simulink model "DA40_Flight_Model"  (R2023a)
settings: Solver=FixedStepAuto  StartTime=Start_Time  StopTime=End_Time  FixedStep=Time_Step  RelTol=1e-3
undefined symbols (not defined in the file or in its folder): BSFC_LUT, dayofyear, Earth, Initial_X, lookaheadDist, PowerFactor_LUT, STGeometry, Vehicle, waypoints, WGS84
libraries: slpidlib x8, simulink_extras x3, aerolibatmos2 x2, mspsensorlib x2, aerolibtransform2 x2, simulink x1, aerolibwind2 x1, uavalgslib x1
(part 2 of 3)

== system DA40_Flight_Model/Truth Model/Control/Subsystem4 ==
  Reference : Inport
  States : Inport  Port=2
  Display : Display
  Display1 : Display
  Display2 : Display
  PID Controller (2DOF) : slpidlib/PID Controller (2DOF)  Controller=PID  Form=Parallel  TimeDomain=Continuous-time  UseExternalTs=off  SampleTime=-1  IntegratorMethod=Forward Euler  FilterMethod=Forward Euler  ControllerParametersSource=internal  P=0  I=1  UseKiTs=off  D=0  N=100  UseFilter=on  b=1  c=1  TunerSelectOption=Transfer Function Based (PID Tuner App)  InitialConditionSource=internal  InitialConditionForIntegrator=0  InitialConditionForFilter=0  DifferentiatorICPrevScaledInput=0  ExternalReset=none  TrackingMode=off  Kt=1  LimitOutput=on  SatLimitsSource=internal  UpperSaturationLimit=1  LowerSaturationLimit=0  LinearizeAsGain=on  AntiWindupMode=none  Kb=1  LimitIntegrator=off  UpperIntegratorSaturationLimit=inf  LowerIntegratorSaturationLimit=-inf  POutMin=[]  POutMax=[]  IOutMin=[]  IOutMax=[]  DOutMin=[]  DOutMax=[]  NOutMin=[]  NOutMax=[]  bOutMin=[]  bOutMax=[]  cOutMin=[]  cOutMax=[]  SumOutMin=[]  SumOutMax=[]  SaturationOutMin=[]  SaturationOutMax=[]  PParamMin=[]  PParamMax=[]  IParamMin=[]  IParamMax=[]  DParamMin=[]  DParamMax=[]  NParamMin=[]  NParamMax=[]  bParamMin=[]  bParamMax=[]  cParamMin=[]  cParamMax=[]  KbParamMin=[]  KbParamMax=[]  KtParamMin=[]  KtParamMax=[]  KbOutMin=[]  KbOutMax=[]  KtOutMin=[]  KtOutMax=[]  IntegratorOutMin=[]  IntegratorOutMax=[]  FilterOutMin=[]  FilterOutMax=[]  SumI1OutMin=[]  SumI1OutMax=[]  SumI2OutMin=[]  SumI2OutMax=[]  SumI3OutMin=[]  SumI3OutMax=[]  SumI4OutMin=[]  SumI4OutMax=[]  SumDOutMin=[]  SumDOutMax=[]  Sum1OutMin=[]  Sum1OutMax=[]  Sum2OutMin=[]  Sum2OutMax=[]  Sum3OutMin=[]  Sum3OutMax=[]  DifferentiatorOutMin=[]  DifferentiatorOutMax=[]  FilterDiffOutCoefMin=[]  FilterDiffOutCoefMax=[]  ReciprocalOutMin=[]  ReciprocalOutMax=[]  SumDenOutMin=[]  SumDenOutMax=[]  SumNumOutMin=[]  SumNumOutMax=[]  DivideOutMin=[]  DivideOutMax=[]  UdiffTsProdOutMin=[]  UdiffTsProdOutMax=[]  NTsProdOutMin=[]  NTsProdOutMax=[]  UintegralTsProdOutMin=[]  UintegralTsProdOutMax=[]  UngainTsProdOutMin=[]  UngainTsProdOutMax=[]  ClampingZeroOutDataTypeStr=Inherit: Inherit via back propagation  ClampingZeroOutMin=[]  ClampingZeroOutMax=[]  FilterDenConstantOutDataTypeStr=Inherit: Inherit via back propagation  FilterDenConstantOutMin=[]  FilterDenConstantOutMax=[]  PCopyOutDataTypeStr=Inherit: Inherit via back propagation  PCopyOutMin=[]  PCopyOutMax=[]  NCopyOutDataTypeStr=Inherit: Inherit via back propagation  NCopyOutMin=[]  NCopyOutMax=[]  IntegratorContinuousStateAttributes=''  IntegratorStateMustResolveToSignalObject=off  IntegratorRTWStateStorageClass=Auto  FilterContinuousStateAttributes=''  FilterStateMustResolveToSignalObject=off  FilterRTWStateStorageClass=Auto  ParallelPVariant=InternalParameters  IdealPVariant=Disabled  IVariant=InternalParameters  DVariant=InternalParameters  bVariant=InternalParameters  cVariant=InternalParameters  IntegratorVariant=Continuous  SatVariant=Enabled  AWVariant=Passthrough  PCopyVariant=Disabled  TRVariant=Disabled  FdbkBlocksVariant=Forward  IdealPFdbkVariant=Disabled  SatFdbkVariant=Disabled  DerivativeFilterVariant=ContFilter  NVariant=InternalParameters  NCopyVariant=Disabled  FilterICVariant=InternalICsFilter  IntegratorICVariant=InternalICs  ExternalResetVariant=Disabled  TRSumVariant=Passthrough  SumFdbkVariant=Disabled  SumVariant=Sum_PID  TsampFilterVariant=InternalTs  TsampNgainVariant=Passthrough  TsampIntegralVariant=Disabled_SignalSpec  ExternalSaturationOutDataTypeStr=Inherit: Same as second input
  Out1 : Outport
  " " : Outport  Port=2
  wires:
  PID Controller (2DOF)/1 -> Display2/1, Out1/1
  [truepropEff] -> Display/1, PID Controller (2DOF)/2
  Reference/1 -> Display1/1, PID Controller (2DOF)/1
  States/1 -> " "/1

== system DA40_Flight_Model/Truth Model/Control/Subsystem5 ==
  Reference : Inport
  States : Inport  Port=2
  Out1 : Outport
  " " : Outport  Port=2
  wires:
  Reference/1 -> Out1/1
  States/1 -> " "/1

== system DA40_Flight_Model/Truth Model/Control/Subsystem6 ==
  Reference : Inport
  States : Inport  Port=2
  Out1 : Outport
  " " : Outport  Port=2
  wires:
  Reference/1 -> Out1/1
  States/1 -> " "/1

== system DA40_Flight_Model/Truth Model/Control/Subsystem7 ==
  Reference : Inport
  States : Inport  Port=2
  Out1 : Outport
  " " : Outport  Port=2
  wires:
  Reference/1 -> Out1/1
  States/1 -> " "/1

== system DA40_Flight_Model/Truth Model/Control/Subsystem8 ==
  Reference : Inport
  States : Inport  Port=2
  Out1 : Outport
  " " : Outport  Port=2
  wires:
  Reference/1 -> Out1/1
  States/1 -> " "/1

== system DA40_Flight_Model/Truth Model/Control/Subsystem9 ==
  Reference : Inport
  States : Inport  Port=2
  Out1 : Outport
  " " : Outport  Port=2
  wires:
  States/1 -> " "/1
  Reference/1 -> Out1/1

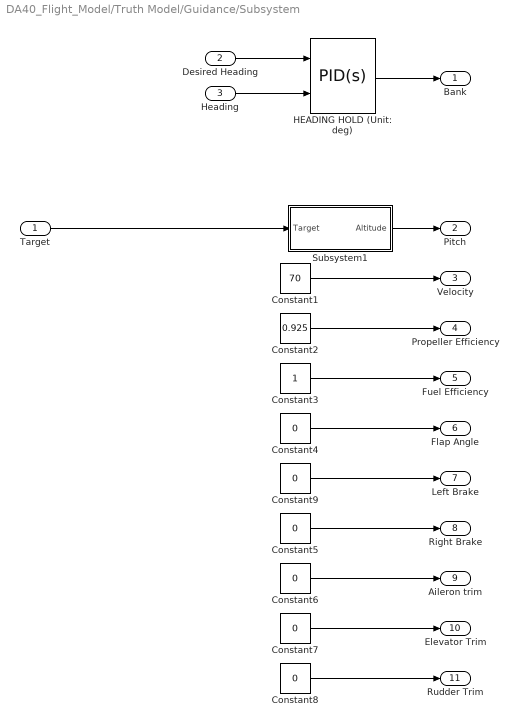
== system DA40_Flight_Model/Truth Model/Guidance/Subsystem ==
  Target : Inport
  Desired Heading : Inport  Port=2
  Heading : Inport  Port=3
  Constant1 : Constant  Value=70
  Constant2 : Constant  Value=0.925
  Constant3 : Constant
  Constant{4..9} (6 alike) : Constant  Value=0
  HEADING HOLD (Unit: deg) : slpidlib/PID Controller (2DOF)  Controller=PID  Form=Parallel  TimeDomain=Continuous-time  UseExternalTs=off  SampleTime=-1  IntegratorMethod=Forward Euler  FilterMethod=Forward Euler  ControllerParametersSource=internal  P=1  I=0.001  UseKiTs=off  D=0  N=100  UseFilter=on  b=1  c=0  TunerSelectOption=Transfer Function Based (PID Tuner App)  InitialConditionSource=internal  InitialConditionForIntegrator=0  InitialConditionForFilter=0  DifferentiatorICPrevScaledInput=0  ExternalReset=none  TrackingMode=off  Kt=1  LimitOutput=on  SatLimitsSource=internal  UpperSaturationLimit=30  LowerSaturationLimit=-30  LinearizeAsGain=on  AntiWindupMode=clamping  Kb=1  LimitIntegrator=off  UpperIntegratorSaturationLimit=inf  LowerIntegratorSaturationLimit=-inf  POutMin=[]  POutMax=[]  IOutMin=[]  IOutMax=[]  DOutMin=[]  DOutMax=[]  NOutMin=[]  NOutMax=[]  bOutMin=[]  bOutMax=[]  cOutMin=[]  cOutMax=[]  SumOutMin=[]  SumOutMax=[]  SaturationOutMin=[]  SaturationOutMax=[]  PParamMin=[]  PParamMax=[]  IParamMin=[]  IParamMax=[]  DParamMin=[]  DParamMax=[]  NParamMin=[]  NParamMax=[]  bParamMin=[]  bParamMax=[]  cParamMin=[]  cParamMax=[]  KbParamMin=[]  KbParamMax=[]  KtParamMin=[]  KtParamMax=[]  KbOutMin=[]  KbOutMax=[]  KtOutMin=[]  KtOutMax=[]  IntegratorOutMin=[]  IntegratorOutMax=[]  FilterOutMin=[]  FilterOutMax=[]  SumI1OutMin=[]  SumI1OutMax=[]  SumI2OutMin=[]  SumI2OutMax=[]  SumI3OutMin=[]  SumI3OutMax=[]  SumI4OutMin=[]  SumI4OutMax=[]  SumDOutMin=[]  SumDOutMax=[]  Sum1OutMin=[]  Sum1OutMax=[]  Sum2OutMin=[]  Sum2OutMax=[]  Sum3OutMin=[]  Sum3OutMax=[]  DifferentiatorOutMin=[]  DifferentiatorOutMax=[]  FilterDiffOutCoefMin=[]  FilterDiffOutCoefMax=[]  ReciprocalOutMin=[]  ReciprocalOutMax=[]  SumDenOutMin=[]  SumDenOutMax=[]  SumNumOutMin=[]  SumNumOutMax=[]  DivideOutMin=[]  DivideOutMax=[]  UdiffTsProdOutMin=[]  UdiffTsProdOutMax=[]  NTsProdOutMin=[]  NTsProdOutMax=[]  UintegralTsProdOutMin=[]  UintegralTsProdOutMax=[]  UngainTsProdOutMin=[]  UngainTsProdOutMax=[]  ClampingZeroOutDataTypeStr=Inherit: Inherit via back propagation  ClampingZeroOutMin=[]  ClampingZeroOutMax=[]  FilterDenConstantOutDataTypeStr=Inherit: Inherit via back propagation  FilterDenConstantOutMin=[]  FilterDenConstantOutMax=[]  PCopyOutDataTypeStr=Inherit: Inherit via back propagation  PCopyOutMin=[]  PCopyOutMax=[]  NCopyOutDataTypeStr=Inherit: Inherit via back propagation  NCopyOutMin=[]  NCopyOutMax=[]  IntegratorContinuousStateAttributes=''  IntegratorStateMustResolveToSignalObject=off  IntegratorRTWStateStorageClass=Auto  FilterContinuousStateAttributes=''  FilterStateMustResolveToSignalObject=off  FilterRTWStateStorageClass=Auto  ParallelPVariant=InternalParameters  IdealPVariant=Disabled  IVariant=InternalParameters  DVariant=InternalParameters  bVariant=InternalParameters  cVariant=InternalParameters  IntegratorVariant=Continuous  SatVariant=Enabled  AWVariant=ContClampingParallel  PCopyVariant=Disabled  TRVariant=Disabled  FdbkBlocksVariant=Forward  IdealPFdbkVariant=Disabled  SatFdbkVariant=Disabled  DerivativeFilterVariant=ContFilter  NVariant=InternalParameters  NCopyVariant=Disabled  FilterICVariant=InternalICsFilter  IntegratorICVariant=InternalICs  ExternalResetVariant=Disabled  TRSumVariant=Passthrough  SumFdbkVariant=Disabled  SumVariant=Sum_PID  TsampFilterVariant=InternalTs  TsampNgainVariant=Passthrough  TsampIntegralVariant=Disabled_SignalSpec  ExternalSaturationOutDataTypeStr=Inherit: Same as second input
  Subsystem1 : Subsystem
  Bank : Outport
  Pitch : Outport  Port=2
  Velocity : Outport  Port=3
  Propeller Efficiency : Outport  Port=4
  Fuel Efficiency : Outport  Port=5
  Flap Angle : Outport  Port=6
  Left Brake : Outport  Port=7
  Right Brake : Outport  Port=8
  Aileron trim : Outport  Port=9
  Elevator Trim : Outport  Port=10
  Rudder Trim : Outport  Port=11
  wires:
  Subsystem1/1(Altitude) -> Pitch/1
  Constant1/1 -> Velocity/1
  Constant2/1 -> Propeller Efficiency/1
  Constant3/1 -> Fuel Efficiency/1
  Constant4/1 -> Flap Angle/1
  Constant9/1 -> Left Brake/1
  Constant5/1 -> Right Brake/1
  Constant6/1 -> Aileron trim/1
  Constant7/1 -> Elevator Trim/1
  Constant8/1 -> Rudder Trim/1
  Desired Heading/1 -> HEADING HOLD (Unit: deg)/1
  Target/1 -> Subsystem1/1(Target)
  HEADING HOLD (Unit: deg)/1 -> Bank/1
  Heading/1 -> HEADING HOLD (Unit: deg)/2

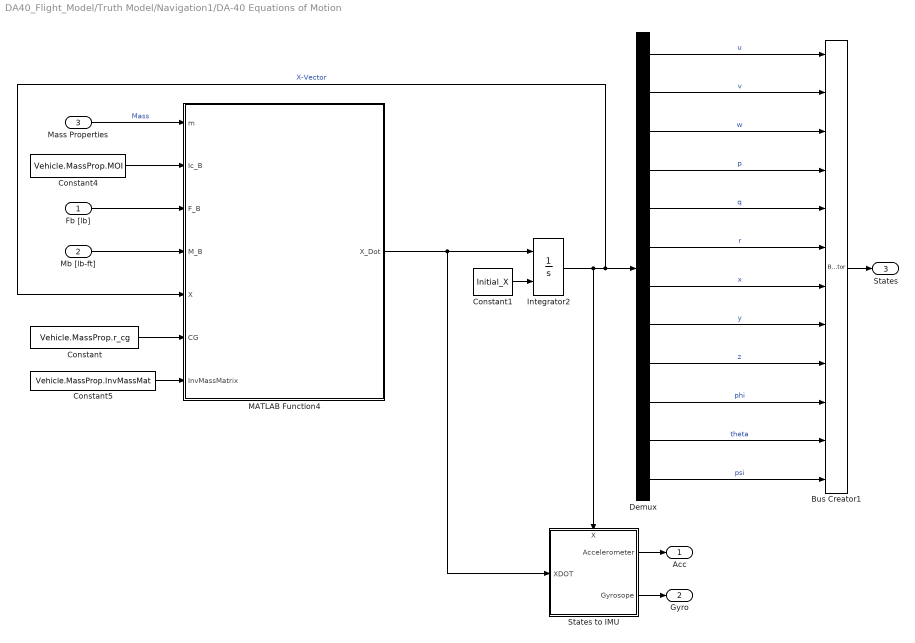
== system DA40_Flight_Model/Truth Model/Navigation1/DA-40 Equations of Motion ==
  Fb [lb] : Inport
  Mb [lb-ft] : Inport  Port=2
  Mass Properties : Inport  Port=3
  Bus Creator1 : BusCreator  Inputs=12
  Constant : Constant  Value=Vehicle.MassProp.r_cg
  Constant1 : Constant  Value=Initial_X
  Constant4 : Constant  Value=Vehicle.MassProp.MOI  VectorParams1D=off
  Constant5 : Constant  Value=Vehicle.MassProp.InvMassMat
  Demux : Demux  Outputs=12
  Integrator2 : Integrator  InitialConditionSource=external
  MATLAB Function4 : MATLAB Function  TreatAsAtomicUnit=on
  States to IMU : Subsystem
      settings: PortSchema="{\"entries\":[{\"content\":{\"sides\":[{\"content\":{\"connectorIds\":[\"In1\"]},\"type\":\"ConnectorPlacement.EquallySpacedRectSide\",\"uuid\":\"70ccec87-9e5d-4668-bab7-5e3830192650\"},{\"content\":{\"connectorIds\":[\"Out1\",\"Out2\"],\"side\":\"RIGHT\"},\"type\":\"ConnectorPlacement.EquallySpacedRectSide\",\"uuid\":\"cc9275bd-5621-4491-a3fb-001b77b42a94\"},{\"content\":{\"connectorIds\":[\"In2\"],\"side\":\"TOP\"},\"type\":\"ConnectorPlacement.EquallySpacedRectSide\",\"uuid\":\"9fc04c5e-8168-4117-852d-b94be052fe47\"}]},\"type\":\"ConnectorPlacement.EquallySpacedConnector\",\"uuid\":\"901299e0-db58-4c82-bff1-da00e9d52dc5\"}],\"packageUris\":[\"http://schema.mathworks.com/mf0/Connector/R2020b\"],\"version\":\"1.0\"}"
  Acc : Outport
  Gyro : Outport  Port=2
  States : Outport  Port=3
  wires:
  Mb [lb-ft]/1 -> MATLAB Function4/4(M_B)
  Fb [lb]/1 -> MATLAB Function4/3(F_B)
  Mass Properties/1 -> MATLAB Function4/1(m)  "Mass"
  Constant4/1 -> MATLAB Function4/2(Ic_B)
  Constant1/1 -> Integrator2/2
  Integrator2/1 -> States to IMU/2(X), MATLAB Function4/5(X), Demux/1  "X-Vector"
  Constant/1 -> MATLAB Function4/6(CG)
  Constant5/1 -> MATLAB Function4/7(InvMassMatrix)
  Demux/1 -> Bus Creator1/1  "u"
  Demux/2 -> Bus Creator1/2  "v"
  Demux/3 -> Bus Creator1/3  "w"
  Demux/4 -> Bus Creator1/4  "p"
  Demux/5 -> Bus Creator1/5  "q"
  Demux/6 -> Bus Creator1/6  "r"
  Demux/7 -> Bus Creator1/7  "x"
  Demux/8 -> Bus Creator1/8  "y"
  Demux/9 -> Bus Creator1/9  "z"
  Demux/10 -> Bus Creator1/10  "phi"
  Demux/11 -> Bus Creator1/11  "theta"
  Demux/12 -> Bus Creator1/12  "psi"
  MATLAB Function4/1(X_Dot) -> States to IMU/1(XDOT), Integrator2/1
  States to IMU/1(Accelerometer) -> Acc/1
  Bus Creator1/1 -> States/1
  States to IMU/2(Gyrosope) -> Gyro/1

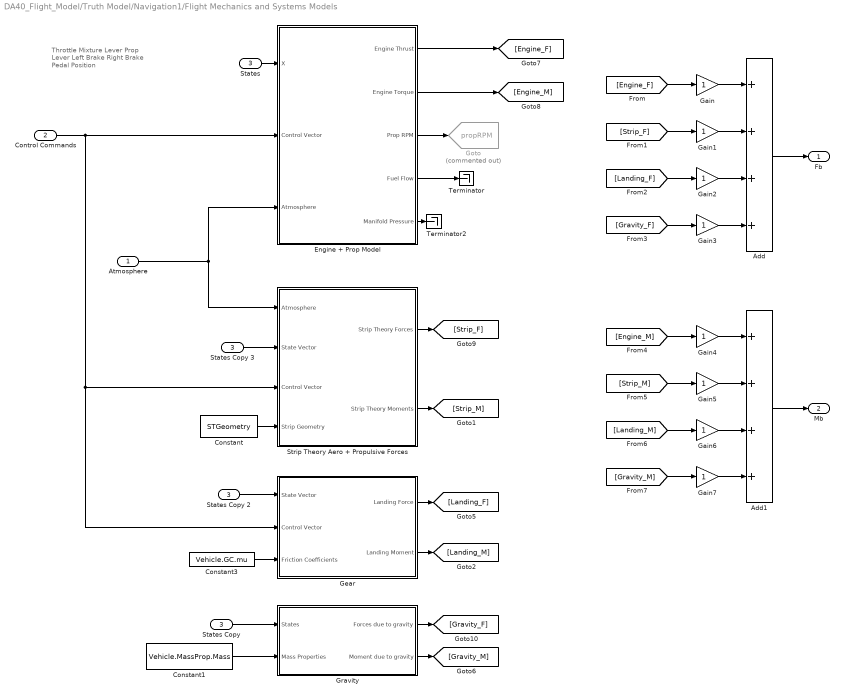
== system DA40_Flight_Model/Truth Model/Navigation1/Flight Mechanics and Systems Models ==
  note: Throttle
      | Mixture Lever
      | Prop Lever
      | Left Brake
      | Right Brake
      | Pedal Position
  Atmosphere : Inport
  Control Commands : Inport  Port=2
  States : Inport  Port=3
  Add : Sum  Inputs=++++
  Add1 : Sum  Inputs=++++
  Constant : Constant  Value=STGeometry
  Constant1 : Constant  Value=Vehicle.MassProp.Mass
  Constant3 : Constant  Value=Vehicle.GC.mu
  Engine + Prop Model : Subsystem
  Gain{,1..7} (8 alike) : Gain
  Gear : Subsystem
  Goto : Goto  Commented=on  GotoTag=propRPM  TagVisibility=global
  Gravity : Subsystem
  States Copy : InportShadow  Port=3
  States Copy 2 : InportShadow  Port=3
  States Copy 3 : InportShadow  Port=3
  Strip Theory Aero + Propulsive Forces : Subsystem
  Terminator : Terminator
  Terminator2 : Terminator
  Fb : Outport
  Mb : Outport  Port=2
  wires:
  States/1 -> Engine + Prop Model/1(X)
  Constant1/1 -> Gravity/2(Mass Properties)
  Constant/1 -> Strip Theory Aero + Propulsive Forces/4(Strip Geometry)
  Engine + Prop Model/5(Manifold Pressure) -> Terminator2/1
  Engine + Prop Model/3(Prop RPM) -> Goto/1
  Constant3/1 -> Gear/3(Friction Coefficients)
  Add1/1 -> Mb/1
  States Copy/1 -> Gravity/1(States)
  States Copy 2/1 -> Gear/1(State Vector)
  States Copy 3/1 -> Strip Theory Aero + Propulsive Forces/2(State Vector)
  Control Commands/1 -> Strip Theory Aero + Propulsive Forces/3(Control Vector), Gear/2(Control Vector), Engine + Prop Model/2(Control Vector)
  Engine + Prop Model/2(Engine Torque) -> [Engine_M]
  Strip Theory Aero + Propulsive Forces/2(Strip Theory Moments) -> [Strip_M]
  Gear/2(Landing Moment) -> [Landing_M]
  Gravity/2(Moment due to gravity) -> [Gravity_M]
  Gravity/1(Forces due to gravity) -> [Gravity_F]
  Gear/1(Landing Force) -> [Landing_F]
  Strip Theory Aero + Propulsive Forces/1(Strip Theory Forces) -> [Strip_F]
  Engine + Prop Model/1(Engine Thrust) -> [Engine_F]
  Add/1 -> Fb/1
  [Engine_F] -> Gain/1
  [Strip_F] -> Gain1/1
  [Landing_F] -> Gain2/1
  [Gravity_F] -> Gain3/1
  [Engine_M] -> Gain4/1
  [Strip_M] -> Gain5/1
  [Landing_M] -> Gain6/1
  [Gravity_M] -> Gain7/1
  Gain/1 -> Add/1
  Gain1/1 -> Add/2
  Gain2/1 -> Add/3
  Gain3/1 -> Add/4
  Gain4/1 -> Add1/1
  Gain5/1 -> Add1/2
  Gain6/1 -> Add1/3
  Gain7/1 -> Add1/4
  Atmosphere/1 -> Strip Theory Aero + Propulsive Forces/1(Atmosphere), Engine + Prop Model/3(Atmosphere)
  Engine + Prop Model/4(Fuel Flow) -> Terminator/1

== system DA40_Flight_Model/Noise Model/Navigation/DA-40 Equations of Motion/States to IMU ==
  XDOT : Inport
  X : Inport  Port=2
  IMU : mspsensorlib/IMU  DispRefFrame=NED  Temperature=25  MagneticFieldNED=[ 27.5550, -2.4169, -16.0849 ]  MagneticFieldENU=[ -2.4169, 27.5550, 16.0849 ]  SeedDouble=67  SimulateUsing=Code generation  AccelParamsMeasurementRange=Inf  AccelParamsResolution=0  AccelParamsConstantBias=[ 0, 0, 0 ]  AccelParamsAxesMisalignment=[ 100, 0, 0; 0, 100, 0; 0, 0, 100 ]  AccelParamsNoiseDensity=[ 0, 0, 0 ]  AccelParamsBiasInstability=[ 0, 0, 0 ]  AccelParamsRandomWalk=[ 0, 0, 0 ]  AccelParamsTemperatureBias=[ 0, 0, 0 ]  AccelParamsTemperatureScaleFactor=[ 0, 0, 0 ]  GyroParamsMeasurementRange=Inf  GyroParamsResolution=0  GyroParamsConstantBias=[ 0, 0, 0 ]  GyroParamsAxesMisalignment=[ 100, 0, 0; 0, 100, 0; 0, 0, 100 ]  GyroParamsAccelerationBias=[ 0, 0, 0 ]  GyroParamsNoiseDensity=[ 0, 0, 0 ]  GyroParamsBiasInstability=[ 0, 0, 0 ]  GyroParamsRandomWalk=[ 0, 0, 0 ]  GyroParamsTemperatureBias=[ 0, 0, 0 ]  GyroParamsTemperatureScaleFactor=[ 0, 0, 0 ]  MagParamsMeasurementRange=Inf  MagParamsResolution=0  MagParamsConstantBias=[ 0, 0, 0 ]  MagParamsAxesMisalignment=[ 100, 0, 0; 0, 100, 0; 0, 0, 100 ]  MagParamsNoiseDensity=[ 0, 0, 0 ]  MagParamsBiasInstability=[ 0, 0, 0 ]  MagParamsRandomWalk=[ 0, 0, 0 ]  MagParamsTemperatureBias=[ 0, 0, 0 ]  MagParamsTemperatureScaleFactor=[ 0, 0, 0 ]
  MATLAB Function : MATLAB Function  TreatAsAtomicUnit=on
  Rate Transition : RateTransition
  Rate Transition1 : RateTransition
  Rate Transition2 : RateTransition
  Terminator : Terminator
  Accelerometer : Outport
  Gyrosope : Outport  Port=2
  wires:
  IMU/3 -> Terminator/1
  IMU/2 -> Gyrosope/1
  IMU/1 -> Accelerometer/1
  X/1 -> MATLAB Function/1(X)
  XDOT/1 -> MATLAB Function/2(XDOT)
  MATLAB Function/1(ACC) -> Rate Transition2/1
  MATLAB Function/2(GYRO) -> Rate Transition1/1
  MATLAB Function/3(DCMBN) -> Rate Transition/1
  Rate Transition/1 -> IMU/3
  Rate Transition1/1 -> IMU/2
  Rate Transition2/1 -> IMU/1

== system DA40_Flight_Model/Noise Model/Navigation/Flight Mechanics and Systems Models/Engine + Prop Model ==
  X : Inport
  Control Vector : Inport  Port=2
  Atmosphere : Inport  Port=3
  Bus Selector : BusSelector  OutputSignals=Throttle,Mixture Lever,Prop Lever
  Subsystem : Subsystem
  Engine Thrust : Outport
  Engine Torque : Outport  Port=2
  Prop RPM : Outport  Port=3  PortDimensions=1
  Fuel Flow : Outport  Port=4  PortDimensions=1
  Manifold Pressure : Outport  Port=5  PortDimensions=1
  wires:
  X/1 -> Subsystem/1(X)
  Subsystem/3(Prop RPM) -> Prop RPM/1
  Subsystem/4(Fuel Flow) -> Fuel Flow/1
  Subsystem/5(Manifold Pressure) -> Manifold Pressure/1
  Control Vector/1 -> Bus Selector/1
  Bus Selector/1 -> Subsystem/2(Throttle Setting)  "<Throttle>"
  Bus Selector/2 -> Subsystem/3(Mix)  "<Mixture Lever>"
  Bus Selector/3 -> Subsystem/4(Prop Pitch)  "<Prop Lever>"
  Atmosphere/1 -> Subsystem/5(Atmosphere)
  Subsystem/2(Engine Torque) -> Engine Torque/1
  Subsystem/1(Engine Thrust) -> Engine Thrust/1

== system DA40_Flight_Model/Noise Model/Navigation/Flight Mechanics and Systems Models/Gear ==
  State Vector : Inport
  Control Vector : Inport  Port=2
  Friction Coefficients : Inport  Port=3
  " " : MATLAB Function  TreatAsAtomicUnit=on
  Bus Selector : BusSelector  OutputSignals=LeftBrake,RightBrake,Pedal Posn
  Mux : Mux  Inputs=3
  Landing Force : Outport
  Landing Moment : Outport  Port=2
  wires:
  Friction Coefficients/1 -> " "/3(mu)
  State Vector/1 -> " "/2(X)
  " "/1(Ground_Forces) -> Landing Force/1
  " "/2(Ground_Moments) -> Landing Moment/1
  Control Vector/1 -> Bus Selector/1
  Mux/1 -> " "/1(U)
  Bus Selector/1 -> Mux/1  "<LeftBrake>"
  Bus Selector/2 -> Mux/2  "<RightBrake>"
  Bus Selector/3 -> Mux/3  "<Pedal Posn>"

== system DA40_Flight_Model/Noise Model/Navigation/Flight Mechanics and Systems Models/Gravity ==
  States : Inport
  Mass Properties : Inport  Port=2
  Constant : Constant  Value=Vehicle.MassProp.r_cg
  MATLAB Function : MATLAB Function  TreatAsAtomicUnit=on
  Forces due to gravity : Outport
  Moment due to gravity : Outport  Port=2
  wires:
  MATLAB Function/1(F_grav_b) -> Forces due to gravity/1
  States/1 -> MATLAB Function/1(X)
  Mass Properties/1 -> MATLAB Function/2(Mass_Properties)
  MATLAB Function/2(M_grav_b) -> Moment due to gravity/1
  Constant/1 -> MATLAB Function/3(CG)

== system DA40_Flight_Model/Noise Model/Navigation/Flight Mechanics and Systems Models/Strip Theory Aero + Propulsive Forces ==
  Atmosphere : Inport
  State Vector : Inport  Port=2
  Control Vector : Inport  Port=3
  Strip Geometry : Inport  Port=4
  Strip_Theory_Modeling : MATLAB Function  TreatAsAtomicUnit=on
  Strip Theory Forces : Outport
  Strip Theory Moments : Outport  Port=2
  wires:
  Atmosphere/1 -> Strip_Theory_Modeling/1(atmos)
  Strip Geometry/1 -> Strip_Theory_Modeling/4(stripGeom)
  Control Vector/1 -> Strip_Theory_Modeling/3(U)
  State Vector/1 -> Strip_Theory_Modeling/2(X)
  Strip_Theory_Modeling/1(Strip_Theory_Forces) -> Strip Theory Forces/1
  Strip_Theory_Modeling/2(Strip_Theory_Moments) -> Strip Theory Moments/1

== system DA40_Flight_Model/Truth Model/Guidance/Subsystem/Subsystem1 ==
  Target : Inport
  Demux : Demux  Outputs=3
  Display : Display
  Gain : Gain  Gain=-1
  Terminator : Terminator
  Terminator1 : Terminator
  Altitude : Outport
  wires:
  Target/1 -> Demux/1
  Demux/3 -> Gain/1
  Demux/2 -> Terminator/1
  Demux/1 -> Terminator1/1
  Gain/1 -> Display/1, Altitude/1

== system DA40_Flight_Model/Truth Model/Navigation1/DA-40 Equations of Motion/States to IMU ==
  XDOT : Inport
  X : Inport  Port=2
  IMU : mspsensorlib/IMU  DispRefFrame=NED  Temperature=25  MagneticFieldNED=[ 27.5550, -2.4169, -16.0849 ]  MagneticFieldENU=[ -2.4169, 27.5550, 16.0849 ]  SeedDouble=67  SimulateUsing=Code generation  AccelParamsMeasurementRange=Inf  AccelParamsResolution=0  AccelParamsConstantBias=[ 0, 0, 0 ]  AccelParamsAxesMisalignment=[ 100, 0, 0; 0, 100, 0; 0, 0, 100 ]  AccelParamsNoiseDensity=[ 0, 0, 0 ]  AccelParamsBiasInstability=[ 0, 0, 0 ]  AccelParamsRandomWalk=[ 0, 0, 0 ]  AccelParamsTemperatureBias=[ 0, 0, 0 ]  AccelParamsTemperatureScaleFactor=[ 0, 0, 0 ]  GyroParamsMeasurementRange=Inf  GyroParamsResolution=0  GyroParamsConstantBias=[ 0, 0, 0 ]  GyroParamsAxesMisalignment=[ 100, 0, 0; 0, 100, 0; 0, 0, 100 ]  GyroParamsAccelerationBias=[ 0, 0, 0 ]  GyroParamsNoiseDensity=[ 0, 0, 0 ]  GyroParamsBiasInstability=[ 0, 0, 0 ]  GyroParamsRandomWalk=[ 0, 0, 0 ]  GyroParamsTemperatureBias=[ 0, 0, 0 ]  GyroParamsTemperatureScaleFactor=[ 0, 0, 0 ]  MagParamsMeasurementRange=Inf  MagParamsResolution=0  MagParamsConstantBias=[ 0, 0, 0 ]  MagParamsAxesMisalignment=[ 100, 0, 0; 0, 100, 0; 0, 0, 100 ]  MagParamsNoiseDensity=[ 0, 0, 0 ]  MagParamsBiasInstability=[ 0, 0, 0 ]  MagParamsRandomWalk=[ 0, 0, 0 ]  MagParamsTemperatureBias=[ 0, 0, 0 ]  MagParamsTemperatureScaleFactor=[ 0, 0, 0 ]
  MATLAB Function : MATLAB Function  TreatAsAtomicUnit=on
  Rate Transition : RateTransition
  Rate Transition1 : RateTransition
  Rate Transition2 : RateTransition
  Terminator : Terminator
  Accelerometer : Outport
  Gyrosope : Outport  Port=2
  wires:
  IMU/3 -> Terminator/1
  IMU/2 -> Gyrosope/1
  IMU/1 -> Accelerometer/1
  X/1 -> MATLAB Function/1(X)
  XDOT/1 -> MATLAB Function/2(XDOT)
  MATLAB Function/1(ACC) -> Rate Transition2/1
  MATLAB Function/2(GYRO) -> Rate Transition1/1
  MATLAB Function/3(DCMBN) -> Rate Transition/1
  Rate Transition/1 -> IMU/3
  Rate Transition1/1 -> IMU/2
  Rate Transition2/1 -> IMU/1

== system DA40_Flight_Model/Truth Model/Navigation1/Flight Mechanics and Systems Models/Engine + Prop Model ==
  X : Inport
  Control Vector : Inport  Port=2
  Atmosphere : Inport  Port=3
  Bus Selector : BusSelector  OutputSignals=Throttle,Mixture Lever,Prop Lever
  Subsystem : Subsystem
  Engine Thrust : Outport
  Engine Torque : Outport  Port=2
  Prop RPM : Outport  Port=3  PortDimensions=1
  Fuel Flow : Outport  Port=4  PortDimensions=1
  Manifold Pressure : Outport  Port=5  PortDimensions=1
  wires:
  X/1 -> Subsystem/1(X)
  Subsystem/3(Prop RPM) -> Prop RPM/1
  Subsystem/4(Fuel Flow) -> Fuel Flow/1
  Subsystem/5(Manifold Pressure) -> Manifold Pressure/1
  Control Vector/1 -> Bus Selector/1
  Bus Selector/1 -> Subsystem/2(Throttle Setting)  "<Throttle>"
  Bus Selector/2 -> Subsystem/3(Mix)  "<Mixture Lever>"
  Bus Selector/3 -> Subsystem/4(Prop Pitch)  "<Prop Lever>"
  Atmosphere/1 -> Subsystem/5(Atmosphere)
  Subsystem/2(Engine Torque) -> Engine Torque/1
  Subsystem/1(Engine Thrust) -> Engine Thrust/1

== system DA40_Flight_Model/Truth Model/Navigation1/Flight Mechanics and Systems Models/Gear ==
  State Vector : Inport
  Control Vector : Inport  Port=2
  Friction Coefficients : Inport  Port=3
  " " : MATLAB Function  TreatAsAtomicUnit=on
  Bus Selector : BusSelector  OutputSignals=LeftBrake,RightBrake,Pedal Posn
  Mux : Mux  Inputs=3
  Landing Force : Outport
  Landing Moment : Outport  Port=2
  wires:
  Friction Coefficients/1 -> " "/3(mu)
  State Vector/1 -> " "/2(X)
  " "/1(Ground_Forces) -> Landing Force/1
  " "/2(Ground_Moments) -> Landing Moment/1
  Control Vector/1 -> Bus Selector/1
  Mux/1 -> " "/1(U)
  Bus Selector/1 -> Mux/1  "<LeftBrake>"
  Bus Selector/2 -> Mux/2  "<RightBrake>"
  Bus Selector/3 -> Mux/3  "<Pedal Posn>"

== system DA40_Flight_Model/Truth Model/Navigation1/Flight Mechanics and Systems Models/Gravity ==
  States : Inport
  Mass Properties : Inport  Port=2
  Constant : Constant  Value=Vehicle.MassProp.r_cg
  MATLAB Function : MATLAB Function  TreatAsAtomicUnit=on
  Forces due to gravity : Outport
  Moment due to gravity : Outport  Port=2
  wires:
  MATLAB Function/1(F_grav_b) -> Forces due to gravity/1
  States/1 -> MATLAB Function/1(X)
  Mass Properties/1 -> MATLAB Function/2(Mass_Properties)
  MATLAB Function/2(M_grav_b) -> Moment due to gravity/1
  Constant/1 -> MATLAB Function/3(CG)

== system DA40_Flight_Model/Truth Model/Navigation1/Flight Mechanics and Systems Models/Strip Theory Aero + Propulsive Forces ==
  Atmosphere : Inport
  State Vector : Inport  Port=2
  Control Vector : Inport  Port=3
  Strip Geometry : Inport  Port=4
  Strip_Theory_Modeling : MATLAB Function  TreatAsAtomicUnit=on
  Strip Theory Forces : Outport
  Strip Theory Moments : Outport  Port=2
  wires:
  Atmosphere/1 -> Strip_Theory_Modeling/1(atmos)
  Strip Geometry/1 -> Strip_Theory_Modeling/4(stripGeom)
  Control Vector/1 -> Strip_Theory_Modeling/3(U)
  State Vector/1 -> Strip_Theory_Modeling/2(X)
  Strip_Theory_Modeling/1(Strip_Theory_Forces) -> Strip Theory Forces/1
  Strip_Theory_Modeling/2(Strip_Theory_Moments) -> Strip Theory Moments/1

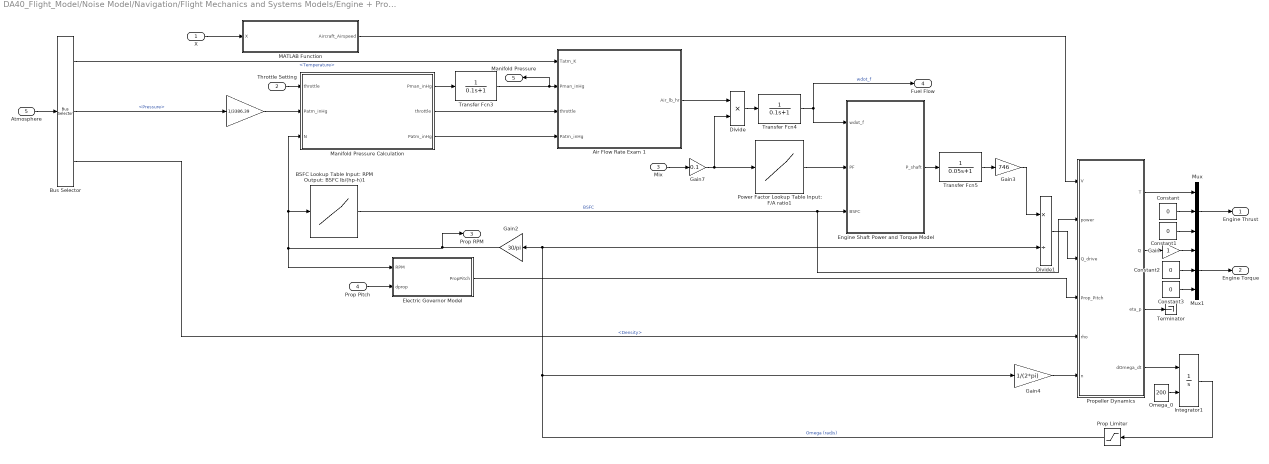
== system DA40_Flight_Model/Noise Model/Navigation/Flight Mechanics and Systems Models/Engine + Prop Model/Subsystem ==
  X : Inport
  Throttle Setting : Inport  Port=2
  Mix : Inport  Port=3
  Prop Pitch : Inport  Port=4
  Atmosphere : Inport  Port=5
  " " : Gain  Gain=1/3386.39
  Air Flow Rate Exam 1 : MATLAB Function  TreatAsAtomicUnit=on
  BSFC Lookup Table Input: RPM Output: BSFC lb/(hp-h)1 : Lookup_n-D  NumberOfTableDimensions=1  BreakpointsForDimension1=BSFC_LUT(1,:)  Table=BSFC_LUT(2,:)  ExtrapMethod=Clip  UseLastTableValue=on  InternalRulePriority=Speed  RndMeth=Simplest
  Bus Selector : BusSelector  OutputSignals=Temperature,Pressure,Density
  Constant{,1..3} (4 alike) : Constant  Value=0
  Divide : Product  Inputs=**
  Divide1 : Product  Inputs=*/
  Electric Governor Model : Subsystem
  Engine Shaft Power and Torque Model : MATLAB Function  TreatAsAtomicUnit=on
  Gain : Gain
  Gain2 : Gain  Gain=30/pi
  Gain3 : Gain  Gain=746
  Gain4 : Gain  Gain=1/(2*pi)
  Gain7 : Gain  Gain=0.1
  Integrator1 : Integrator  InitialConditionSource=external
  MATLAB Function : MATLAB Function  TreatAsAtomicUnit=on
  Manifold Pressure Calculation : MATLAB Function  TreatAsAtomicUnit=on
  Mux : Mux  Inputs=3
  Mux1 : Mux  Inputs=3
  Omega_0 : Constant  Value=200
  Power Factor Lookup Table Input: F/A ratio1 : Lookup_n-D  NumberOfTableDimensions=1  BreakpointsForDimension1=PowerFactor_LUT(1,:)  Table=PowerFactor_LUT(2,:)  ExtrapMethod=Clip  UseLastTableValue=on  InternalRulePriority=Speed  RndMeth=Simplest
  Prop Limiter : Saturate  UpperLimit=320  LowerLimit=0
  Propeller Dynamics : MATLAB Function  TreatAsAtomicUnit=on
  Terminator : Terminator
  Transfer Fcn3 : TransferFcn  Denominator=[0.1 1]
  Transfer Fcn4 : TransferFcn  Denominator=[0.1 1]
  Transfer Fcn5 : TransferFcn  Denominator=[0.05 1]
  Engine Thrust : Outport
  Engine Torque : Outport  Port=2
  Prop RPM : Outport  Port=3  PortDimensions=1
  Fuel Flow : Outport  Port=4  PortDimensions=1
  Manifold Pressure : Outport  Port=5  PortDimensions=1
  wires:
  Transfer Fcn4/1 -> Engine Shaft Power and Torque Model/1(wdot_f), Fuel Flow/1  "wdot_f"
  Constant2/1 -> Mux1/2
  Propeller Dynamics/4(dOmega_dt) -> Integrator1/1
  Mux/1 -> Engine Thrust/1
  Gain2/1 -> Prop RPM/1, Electric Governor Model/1(RPM), BSFC Lookup Table Input: RPM Output: BSFC lb/(hp-h)1/1, Manifold Pressure Calculation/3(N)
  Electric Governor Model/1(PropPitch) -> Propeller Dynamics/4(Prop_Pitch)
  Divide/1 -> Transfer Fcn4/1
  Propeller Dynamics/3(eta_p) -> Terminator/1
  Constant/1 -> Mux/2
  Gain4/1 -> Propeller Dynamics/6(n)
  Mix/1 -> Gain7/1
  Bus Selector/3 -> Propeller Dynamics/5(rho)  "<Density>"
  Manifold Pressure Calculation/3(Patm_inHg) -> Air Flow Rate Exam 1/4(Patm_inHg)
  BSFC Lookup Table Input: RPM Output: BSFC lb/(hp-h)1/1 -> Propeller Dynamics/2(power), Engine Shaft Power and Torque Model/3(BSFC)  "BSFC"
  Manifold Pressure Calculation/2(throttle) -> Air Flow Rate Exam 1/3(throttle)
  Prop Limiter/1 -> Divide1/2, Gain2/1, Gain4/1  "Omega (rad/s)"
  Propeller Dynamics/1(T) -> Mux/1
  Engine Shaft Power and Torque Model/1(P_shaft) -> Transfer Fcn5/1
  Omega_0/1 -> Integrator1/2
  Constant3/1 -> Mux1/3
  Transfer Fcn3/1 -> Manifold Pressure/1, Air Flow Rate Exam 1/2(Pman_inHg)
  Power Factor Lookup Table Input: F/A ratio1/1 -> Engine Shaft Power and Torque Model/2(PF)
  X/1 -> MATLAB Function/1(X)
  Gain3/1 -> Divide1/1
  Prop Pitch/1 -> Electric Governor Model/2(dprop)
  Transfer Fcn5/1 -> Gain3/1
  Propeller Dynamics/2(Q) -> Gain/1
  Mux1/1 -> Engine Torque/1
  Gain/1 -> Mux1/1
  Divide1/1 -> Propeller Dynamics/3(Q_drive)
  Manifold Pressure Calculation/1(Pman_inHg) -> Transfer Fcn3/1
  Gain7/1 -> Power Factor Lookup Table Input: F/A ratio1/1, Divide/2
  MATLAB Function/1(Aircraft_Airspeed) -> Propeller Dynamics/1(V)
  Throttle Setting/1 -> Manifold Pressure Calculation/1("throttle ")
  " "/1 -> Manifold Pressure Calculation/2("Patm_inHg ")
  Constant1/1 -> Mux/3
  Atmosphere/1 -> Bus Selector/1
  Bus Selector/1 -> Air Flow Rate Exam 1/1(Tatm_K)  "<Temperature>"
  Bus Selector/2 -> " "/1  "<Pressure>"
  Air Flow Rate Exam 1/1(Air_lb_hr) -> Divide/1
  Integrator1/1 -> Prop Limiter/1

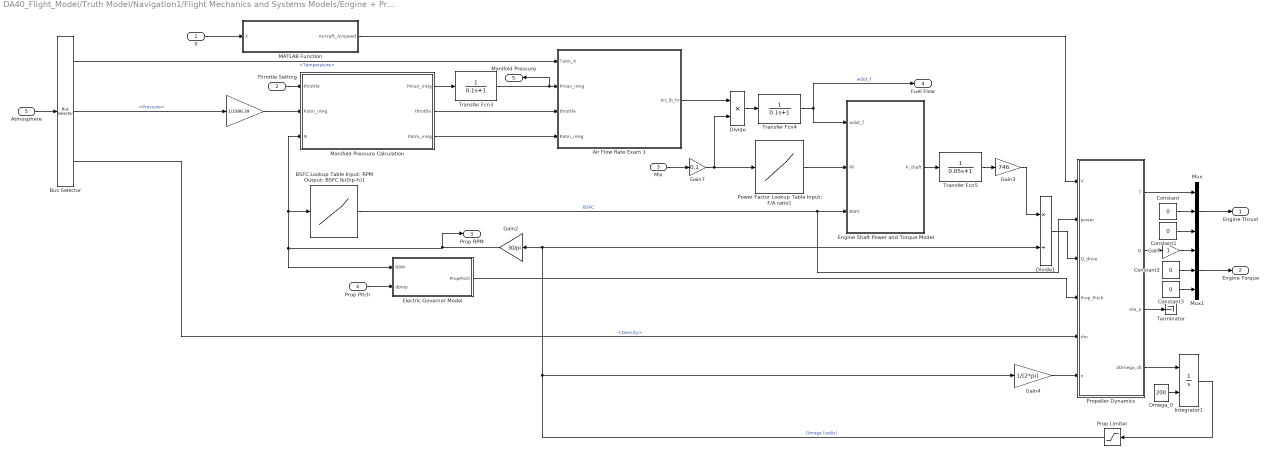
== system DA40_Flight_Model/Truth Model/Navigation1/Flight Mechanics and Systems Models/Engine + Prop Model/Subsystem ==
  X : Inport
  Throttle Setting : Inport  Port=2
  Mix : Inport  Port=3
  Prop Pitch : Inport  Port=4
  Atmosphere : Inport  Port=5
  " " : Gain  Gain=1/3386.39
  Air Flow Rate Exam 1 : MATLAB Function  TreatAsAtomicUnit=on
  BSFC Lookup Table Input: RPM Output: BSFC lb/(hp-h)1 : Lookup_n-D  NumberOfTableDimensions=1  BreakpointsForDimension1=BSFC_LUT(1,:)  Table=BSFC_LUT(2,:)  ExtrapMethod=Clip  UseLastTableValue=on  InternalRulePriority=Speed  RndMeth=Simplest
  Bus Selector : BusSelector  OutputSignals=Temperature,Pressure,Density
  Constant{,1..3} (4 alike) : Constant  Value=0
  Divide : Product  Inputs=**
  Divide1 : Product  Inputs=*/
  Electric Governor Model : Subsystem
  Engine Shaft Power and Torque Model : MATLAB Function  TreatAsAtomicUnit=on
  Gain : Gain
  Gain2 : Gain  Gain=30/pi
  Gain3 : Gain  Gain=746
  Gain4 : Gain  Gain=1/(2*pi)
  Gain7 : Gain  Gain=0.1
  Integrator1 : Integrator  InitialConditionSource=external
  MATLAB Function : MATLAB Function  TreatAsAtomicUnit=on
  Manifold Pressure Calculation : MATLAB Function  TreatAsAtomicUnit=on
  Mux : Mux  Inputs=3
  Mux1 : Mux  Inputs=3
  Omega_0 : Constant  Value=200
  Power Factor Lookup Table Input: F/A ratio1 : Lookup_n-D  NumberOfTableDimensions=1  BreakpointsForDimension1=PowerFactor_LUT(1,:)  Table=PowerFactor_LUT(2,:)  ExtrapMethod=Clip  UseLastTableValue=on  InternalRulePriority=Speed  RndMeth=Simplest
  Prop Limiter : Saturate  UpperLimit=320  LowerLimit=0
  Propeller Dynamics : MATLAB Function  TreatAsAtomicUnit=on
  Terminator : Terminator
  Transfer Fcn3 : TransferFcn  Denominator=[0.1 1]
  Transfer Fcn4 : TransferFcn  Denominator=[0.1 1]
  Transfer Fcn5 : TransferFcn  Denominator=[0.05 1]
  Engine Thrust : Outport
  Engine Torque : Outport  Port=2
  Prop RPM : Outport  Port=3  PortDimensions=1
  Fuel Flow : Outport  Port=4  PortDimensions=1
  Manifold Pressure : Outport  Port=5  PortDimensions=1
  wires:
  Transfer Fcn4/1 -> Engine Shaft Power and Torque Model/1(wdot_f), Fuel Flow/1  "wdot_f"
  Constant2/1 -> Mux1/2
  Propeller Dynamics/4(dOmega_dt) -> Integrator1/1
  Mux/1 -> Engine Thrust/1
  Gain2/1 -> Prop RPM/1, Electric Governor Model/1(RPM), BSFC Lookup Table Input: RPM Output: BSFC lb/(hp-h)1/1, Manifold Pressure Calculation/3(N)
  Electric Governor Model/1(PropPitch) -> Propeller Dynamics/4(Prop_Pitch)
  Divide/1 -> Transfer Fcn4/1
  Propeller Dynamics/3(eta_p) -> Terminator/1
  Constant/1 -> Mux/2
  Gain4/1 -> Propeller Dynamics/6(n)
  Mix/1 -> Gain7/1
  Bus Selector/3 -> Propeller Dynamics/5(rho)  "<Density>"
  Manifold Pressure Calculation/3(Patm_inHg) -> Air Flow Rate Exam 1/4(Patm_inHg)
  BSFC Lookup Table Input: RPM Output: BSFC lb/(hp-h)1/1 -> Propeller Dynamics/2(power), Engine Shaft Power and Torque Model/3(BSFC)  "BSFC"
  Manifold Pressure Calculation/2(throttle) -> Air Flow Rate Exam 1/3(throttle)
  Prop Limiter/1 -> Divide1/2, Gain2/1, Gain4/1  "Omega (rad/s)"
  Propeller Dynamics/1(T) -> Mux/1
  Engine Shaft Power and Torque Model/1(P_shaft) -> Transfer Fcn5/1
  Omega_0/1 -> Integrator1/2
  Constant3/1 -> Mux1/3
  Transfer Fcn3/1 -> Manifold Pressure/1, Air Flow Rate Exam 1/2(Pman_inHg)
  Power Factor Lookup Table Input: F/A ratio1/1 -> Engine Shaft Power and Torque Model/2(PF)
  X/1 -> MATLAB Function/1(X)
  Gain3/1 -> Divide1/1
  Prop Pitch/1 -> Electric Governor Model/2(dprop)
  Transfer Fcn5/1 -> Gain3/1
  Propeller Dynamics/2(Q) -> Gain/1
  Mux1/1 -> Engine Torque/1
  Gain/1 -> Mux1/1
  Divide1/1 -> Propeller Dynamics/3(Q_drive)
  Manifold Pressure Calculation/1(Pman_inHg) -> Transfer Fcn3/1
  Gain7/1 -> Power Factor Lookup Table Input: F/A ratio1/1, Divide/2
  MATLAB Function/1(Aircraft_Airspeed) -> Propeller Dynamics/1(V)
  Throttle Setting/1 -> Manifold Pressure Calculation/1("throttle ")
  " "/1 -> Manifold Pressure Calculation/2("Patm_inHg ")
  Constant1/1 -> Mux/3
  Atmosphere/1 -> Bus Selector/1
  Bus Selector/1 -> Air Flow Rate Exam 1/1(Tatm_K)  "<Temperature>"
  Bus Selector/2 -> " "/1  "<Pressure>"
  Air Flow Rate Exam 1/1(Air_lb_hr) -> Divide/1
  Integrator1/1 -> Prop Limiter/1

== system DA40_Flight_Model/Noise Model/Navigation/Flight Mechanics and Systems Models/Engine + Prop Model/Subsystem/Electric Governor Model ==
  RPM : Inport
  dprop : Inport  Port=2
  Constant : Constant  Value=0
  DESIRED RPM : MATLABFcn  MATLABFcn=800 + 2000 * u
  Initial Blade Pitch : Constant  Value=5
  PID Controller (2DOF) : slpidlib/PID Controller (2DOF)  Controller=PID  Form=Parallel  TimeDomain=Continuous-time  UseExternalTs=off  SampleTime=-1  IntegratorMethod=Forward Euler  FilterMethod=Forward Euler  ControllerParametersSource=internal  P=-.08  I=-0.01  UseKiTs=off  D=0  N=100  UseFilter=on  b=1  c=0  TunerSelectOption=Transfer Function Based (PID Tuner App)  InitialConditionSource=external  InitialConditionForIntegrator=0  InitialConditionForFilter=0  DifferentiatorICPrevScaledInput=0  ExternalReset=none  TrackingMode=off  Kt=1  LimitOutput=on  SatLimitsSource=internal  UpperSaturationLimit=26  LowerSaturationLimit=10  LinearizeAsGain=on  AntiWindupMode=clamping  Kb=1  LimitIntegrator=off  UpperIntegratorSaturationLimit=inf  LowerIntegratorSaturationLimit=-inf  POutMin=[]  POutMax=[]  IOutMin=[]  IOutMax=[]  DOutMin=[]  DOutMax=[]  NOutMin=[]  NOutMax=[]  bOutMin=[]  bOutMax=[]  cOutMin=[]  cOutMax=[]  SumOutMin=[]  SumOutMax=[]  SaturationOutMin=[]  SaturationOutMax=[]  PParamMin=[]  PParamMax=[]  IParamMin=[]  IParamMax=[]  DParamMin=[]  DParamMax=[]  NParamMin=[]  NParamMax=[]  bParamMin=[]  bParamMax=[]  cParamMin=[]  cParamMax=[]  KbParamMin=[]  KbParamMax=[]  KtParamMin=[]  KtParamMax=[]  KbOutMin=[]  KbOutMax=[]  KtOutMin=[]  KtOutMax=[]  IntegratorOutMin=[]  IntegratorOutMax=[]  FilterOutMin=[]  FilterOutMax=[]  SumI1OutMin=[]  SumI1OutMax=[]  SumI2OutMin=[]  SumI2OutMax=[]  SumI3OutMin=[]  SumI3OutMax=[]  SumI4OutMin=[]  SumI4OutMax=[]  SumDOutMin=[]  SumDOutMax=[]  Sum1OutMin=[]  Sum1OutMax=[]  Sum2OutMin=[]  Sum2OutMax=[]  Sum3OutMin=[]  Sum3OutMax=[]  DifferentiatorOutMin=[]  DifferentiatorOutMax=[]  FilterDiffOutCoefMin=[]  FilterDiffOutCoefMax=[]  ReciprocalOutMin=[]  ReciprocalOutMax=[]  SumDenOutMin=[]  SumDenOutMax=[]  SumNumOutMin=[]  SumNumOutMax=[]  DivideOutMin=[]  DivideOutMax=[]  UdiffTsProdOutMin=[]  UdiffTsProdOutMax=[]  NTsProdOutMin=[]  NTsProdOutMax=[]  UintegralTsProdOutMin=[]  UintegralTsProdOutMax=[]  UngainTsProdOutMin=[]  UngainTsProdOutMax=[]  ClampingZeroOutDataTypeStr=Inherit: Inherit via back propagation  ClampingZeroOutMin=[]  ClampingZeroOutMax=[]  FilterDenConstantOutDataTypeStr=Inherit: Inherit via back propagation  FilterDenConstantOutMin=[]  FilterDenConstantOutMax=[]  PCopyOutDataTypeStr=Inherit: Inherit via back propagation  PCopyOutMin=[]  PCopyOutMax=[]  NCopyOutDataTypeStr=Inherit: Inherit via back propagation  NCopyOutMin=[]  NCopyOutMax=[]  IntegratorContinuousStateAttributes=''  IntegratorStateMustResolveToSignalObject=off  IntegratorRTWStateStorageClass=Auto  FilterContinuousStateAttributes=''  FilterStateMustResolveToSignalObject=off  FilterRTWStateStorageClass=Auto  ParallelPVariant=InternalParameters  IdealPVariant=Disabled  IVariant=InternalParameters  DVariant=InternalParameters  bVariant=InternalParameters  cVariant=InternalParameters  IntegratorVariant=Continuous  SatVariant=Enabled  AWVariant=ContClampingParallel  PCopyVariant=Disabled  TRVariant=Disabled  FdbkBlocksVariant=Forward  IdealPFdbkVariant=Disabled  SatFdbkVariant=Disabled  DerivativeFilterVariant=ContFilter  NVariant=InternalParameters  NCopyVariant=Disabled  FilterICVariant=ExternalICs  IntegratorICVariant=ExternalICs  ExternalResetVariant=Disabled  TRSumVariant=Passthrough  SumFdbkVariant=Disabled  SumVariant=Sum_PID  TsampFilterVariant=InternalTs  TsampNgainVariant=Passthrough  TsampIntegralVariant=Disabled_SignalSpec  ExternalSaturationOutDataTypeStr=Inherit: Same as second input
  Saturation : Saturate  UpperLimit=2650  LowerLimit=800
  PropPitch : Outport
  wires:
  dprop/1 -> DESIRED RPM/1
  PID Controller (2DOF)/1 -> PropPitch/1
  Constant/1 -> PID Controller (2DOF)/4
  Initial Blade Pitch/1 -> PID Controller (2DOF)/3
  DESIRED RPM/1 -> Saturation/1
  RPM/1 -> PID Controller (2DOF)/2
  Saturation/1 -> PID Controller (2DOF)/1

== system DA40_Flight_Model/Truth Model/Navigation1/Flight Mechanics and Systems Models/Engine + Prop Model/Subsystem/Electric Governor Model ==
  RPM : Inport
  dprop : Inport  Port=2
  Constant : Constant  Value=0
  DESIRED RPM : MATLABFcn  MATLABFcn=800 + 2000 * u
  Initial Blade Pitch : Constant  Value=5
  PID Controller (2DOF) : slpidlib/PID Controller (2DOF)  Controller=PID  Form=Parallel  TimeDomain=Continuous-time  UseExternalTs=off  SampleTime=-1  IntegratorMethod=Forward Euler  FilterMethod=Forward Euler  ControllerParametersSource=internal  P=-.08  I=-0.01  UseKiTs=off  D=0  N=100  UseFilter=on  b=1  c=0  TunerSelectOption=Transfer Function Based (PID Tuner App)  InitialConditionSource=external  InitialConditionForIntegrator=0  InitialConditionForFilter=0  DifferentiatorICPrevScaledInput=0  ExternalReset=none  TrackingMode=off  Kt=1  LimitOutput=on  SatLimitsSource=internal  UpperSaturationLimit=26  LowerSaturationLimit=10  LinearizeAsGain=on  AntiWindupMode=clamping  Kb=1  LimitIntegrator=off  UpperIntegratorSaturationLimit=inf  LowerIntegratorSaturationLimit=-inf  POutMin=[]  POutMax=[]  IOutMin=[]  IOutMax=[]  DOutMin=[]  DOutMax=[]  NOutMin=[]  NOutMax=[]  bOutMin=[]  bOutMax=[]  cOutMin=[]  cOutMax=[]  SumOutMin=[]  SumOutMax=[]  SaturationOutMin=[]  SaturationOutMax=[]  PParamMin=[]  PParamMax=[]  IParamMin=[]  IParamMax=[]  DParamMin=[]  DParamMax=[]  NParamMin=[]  NParamMax=[]  bParamMin=[]  bParamMax=[]  cParamMin=[]  cParamMax=[]  KbParamMin=[]  KbParamMax=[]  KtParamMin=[]  KtParamMax=[]  KbOutMin=[]  KbOutMax=[]  KtOutMin=[]  KtOutMax=[]  IntegratorOutMin=[]  IntegratorOutMax=[]  FilterOutMin=[]  FilterOutMax=[]  SumI1OutMin=[]  SumI1OutMax=[]  SumI2OutMin=[]  SumI2OutMax=[]  SumI3OutMin=[]  SumI3OutMax=[]  SumI4OutMin=[]  SumI4OutMax=[]  SumDOutMin=[]  SumDOutMax=[]  Sum1OutMin=[]  Sum1OutMax=[]  Sum2OutMin=[]  Sum2OutMax=[]  Sum3OutMin=[]  Sum3OutMax=[]  DifferentiatorOutMin=[]  DifferentiatorOutMax=[]  FilterDiffOutCoefMin=[]  FilterDiffOutCoefMax=[]  ReciprocalOutMin=[]  ReciprocalOutMax=[]  SumDenOutMin=[]  SumDenOutMax=[]  SumNumOutMin=[]  SumNumOutMax=[]  DivideOutMin=[]  DivideOutMax=[]  UdiffTsProdOutMin=[]  UdiffTsProdOutMax=[]  NTsProdOutMin=[]  NTsProdOutMax=[]  UintegralTsProdOutMin=[]  UintegralTsProdOutMax=[]  UngainTsProdOutMin=[]  UngainTsProdOutMax=[]  ClampingZeroOutDataTypeStr=Inherit: Inherit via back propagation  ClampingZeroOutMin=[]  ClampingZeroOutMax=[]  FilterDenConstantOutDataTypeStr=Inherit: Inherit via back propagation  FilterDenConstantOutMin=[]  FilterDenConstantOutMax=[]  PCopyOutDataTypeStr=Inherit: Inherit via back propagation  PCopyOutMin=[]  PCopyOutMax=[]  NCopyOutDataTypeStr=Inherit: Inherit via back propagation  NCopyOutMin=[]  NCopyOutMax=[]  IntegratorContinuousStateAttributes=''  IntegratorStateMustResolveToSignalObject=off  IntegratorRTWStateStorageClass=Auto  FilterContinuousStateAttributes=''  FilterStateMustResolveToSignalObject=off  FilterRTWStateStorageClass=Auto  ParallelPVariant=InternalParameters  IdealPVariant=Disabled  IVariant=InternalParameters  DVariant=InternalParameters  bVariant=InternalParameters  cVariant=InternalParameters  IntegratorVariant=Continuous  SatVariant=Enabled  AWVariant=ContClampingParallel  PCopyVariant=Disabled  TRVariant=Disabled  FdbkBlocksVariant=Forward  IdealPFdbkVariant=Disabled  SatFdbkVariant=Disabled  DerivativeFilterVariant=ContFilter  NVariant=InternalParameters  NCopyVariant=Disabled  FilterICVariant=ExternalICs  IntegratorICVariant=ExternalICs  ExternalResetVariant=Disabled  TRSumVariant=Passthrough  SumFdbkVariant=Disabled  SumVariant=Sum_PID  TsampFilterVariant=InternalTs  TsampNgainVariant=Passthrough  TsampIntegralVariant=Disabled_SignalSpec  ExternalSaturationOutDataTypeStr=Inherit: Same as second input
  Saturation : Saturate  UpperLimit=2650  LowerLimit=800
  PropPitch : Outport
  wires:
  dprop/1 -> DESIRED RPM/1
  PID Controller (2DOF)/1 -> PropPitch/1
  Constant/1 -> PID Controller (2DOF)/4
  Initial Blade Pitch/1 -> PID Controller (2DOF)/3
  DESIRED RPM/1 -> Saturation/1
  RPM/1 -> PID Controller (2DOF)/2
  Saturation/1 -> PID Controller (2DOF)/1

== matlab function DA40_Flight_Model/Truth Model/Navigation1/Flight Mechanics and Systems Models/Engine + Prop Model/Subsystem/MATLAB Function ==
  data: X input; Aircraft_Airspeed output
function Aircraft_Airspeed = Calc_AC_Speed(X)
Aircraft_Airspeed = norm(X(1:3));
end

== matlab function DA40_Flight_Model/Truth Model/Navigation1/Flight Mechanics and Systems Models/Engine + Prop Model/Subsystem/Manifold Pressure Calculation ==
  data: throttle input; Patm_inHg input; N input; Pman_inHg output; throttle output; Patm_inHg output
function [Pman_inHg,throttle,Patm_inHg]  = fcn(throttle,Patm_inHg,N)

Pman_inHg = Patm_inHg + (0.007*throttle - 0.0086)*N;

end

== matlab function DA40_Flight_Model/Truth Model/Navigation1/Flight Mechanics and Systems Models/Engine + Prop Model/Subsystem/Propeller Dynamics ==
  data: V input; power input; Q_drive input size=1; Prop_Pitch input; rho input; n input; T output; Q output; eta_p output size=1; dOmega_dt output
function [T,Q,eta_p,dOmega_dt] = VarP_PropDynamics(V,power, Q_drive,Prop_Pitch,rho,n)

T = 0;
Q = 0;
eta_p = 0;
dOmega_dt = 0;

coder.extrinsic('griddedInterpolant')
coder.extrinsic('CTCQPropeff')

[T,Q,eta_p,dOmega_dt] = CTCQPropeff(Prop_Pitch,power,Q_drive,rho,V,n,[]);

end
